simulink model "task1_4"  (R2015b)
settings: Solver=ode45  StartTime=tstart  StopTime=tstop  RelTol=1e-3
values from neighbouring files (symbols this model uses):
  c = 0    [NonLinearAnalysis.m]    (also in Run_Delta_R_Sim.m; analyse_lin_dynamics.m; analyse_steadystate.m; analyse_ulin_dynamics kopi.m)
  delta_max = 0.436332312999    [Yaw and Yaw-rate controller.mat]    (also in Yaw_NonLin_controller.mat; Yaw_PID_controller.mat; run_task1_4.m = deg2rad(25))
  IN = i    [run_task1_4.m]
  K = 0.0516730310612    [Heading_model.mat]    (also in Nomoto2_curvefitting.mat = 0.0627494534487; analyse_controller.m = place(A,B,P); analyse_lin_dynamics.m = x(2); analyse_ulin_dynamics kopi.m = x(2))
  k_b0 = 0.009    [Yaw and Yaw-rate controller.mat]    (also in Yaw_NonLin_controller.mat; Yaw_PID_controller.mat; run_task1_4.m)
  k_b1 = 3.06871796591e-14    [Yaw and Yaw-rate controller.mat]    (also in Yaw_NonLin_controller.mat = 1.2654213265e-10; run_task1_4.m = b_2(2))
  k_b2 = 291.893339409    [Yaw and Yaw-rate controller.mat]    (also in Yaw_NonLin_controller.mat = 288.459058131; run_task1_4.m = b_2(3))
  k_b3 = 1233422.7042    [Yaw and Yaw-rate controller.mat]    (also in Yaw_NonLin_controller.mat = 1209648.75063; run_task1_4.m = b_2(1))
  kd_psi = 3    [Yaw and Yaw-rate controller.mat]    (also in Yaw_NonLin_controller.mat; Yaw_PID_controller.mat = 300; run_task1_4.m = 300)
  ki_psi = 2e-05    [Yaw and Yaw-rate controller.mat]    (also in Yaw_NonLin_controller.mat; Yaw_PID_controller.mat = 0.8; run_task1_4.m = 0.8)
  kp_psi = 0.015    [Yaw and Yaw-rate controller.mat]    (also in Yaw_NonLin_controller.mat; Yaw_PID_controller.mat = 90; run_task1_4.m = 90)
  n_c = 7.3    [run_task1_4.m]
  psi0 = 0    [NonLinearAnalysis.m]    (also in Run_Delta_R_Sim.m; analyse_lin_dynamics.m; analyse_steadystate.m; analyse_ulin_dynamics kopi.m)
  r0 = 0    [NonLinearAnalysis.m]    (also in Run_Delta_R_Sim.m; analyse_lin_dynamics.m; analyse_steadystate.m; analyse_ulin_dynamics kopi.m)
  T1 = 147.34337747    [Heading_model.mat]    (also in Nomoto2_curvefitting.mat = 53.2599278148; analyse_controller.m = 130; analyse_lin_dynamics.m = x(1); analyse_ulin_dynamics kopi.m = x(1))
  T2 = 157.062217136    [Heading_model.mat]    (also in Nomoto2_curvefitting.mat = 67.2891048935; analyse_controller.m = 150; analyse_lin_dynamics.m = x(2); analyse_ulin_dynamics kopi.m = x(2))
  T3 = 252.073612676    [Heading_model.mat]    (also in Nomoto2_curvefitting.mat = 168; analyse_controller.m = 320; analyse_lin_dynamics.m = x(3); analyse_ulin_dynamics kopi.m = x(3))
  tsamp = 10    [NonLinearAnalysis.m]    (also in analyse_lin_dynamics.m; analyse_steadystate.m; analyse_ulin_dynamics kopi.m; analyse_ulin_dynamics.m)
  v0 = [6.63 0]'    [NonLinearAnalysis.m]    (also in Run_Delta_R_Sim.m; analyse_lin_dynamics.m; analyse_steadystate.m; analyse_ulin_dynamics kopi.m)
  w_psi = 0.04    [Yaw and Yaw-rate controller.mat]    (also in Yaw_NonLin_controller.mat; Yaw_PID_controller.mat = 0.05; run_task1_4.m = 0.05)
undefined symbols (not defined in the file or in its folder): msfartoystyring
undefined symbols (not defined in the file): p0
settings Model: ExtModeAutoUpdateStatusClock=off  Creator=christh  LastModifiedBy=Erik
settings DataIOCC: SaveFormat=Array  SignalLoggingSaveFormat=ModelDataLogs
settings OptimizationCC: ExpressionDepthLimit=2147483647  InitFltsAndDblsToZero=on
settings DebuggingCC: UnderspecifiedInitializationDetection=Classic  MergeDetectMultiDrivingBlocksExec=none  SolverPrmCheckMsg=warning  FcnCallInpInsideContextMsg=UseLocalSettings  StateNameClashWarn=warning
settings HardwareCC: ProdBitPerPointer=32  ProdLargestAtomicFloat=None  ProdIntDivRoundTo=Undefined  ProdEndianess=Unspecified  ProdWordSize=32  ProdHWDeviceType=32-bit Generic
settings GRTTargetCC: GeneratePreprocessorConditionals=Disable all  CombineOutputUpdateFcns=off  GRTInterface=on
settings ConfigComp: CovModelRefEnable=Off

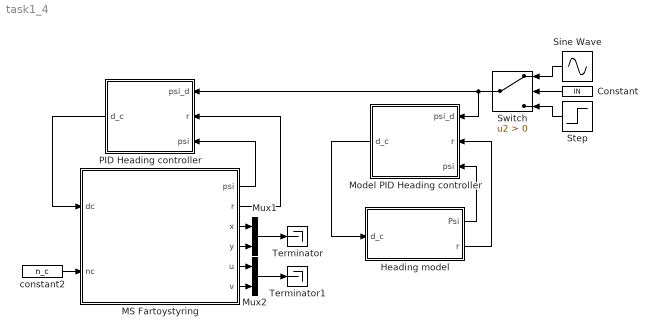
== system task1_4 ==
  Constant : Constant  Value=IN
  Heading model : Subsystem
  MS Fartoystyring : Subsystem  mask(MS Fartoystyring for Assignment 3 G&C){x0=p0(1), y0=p0(2), u0=v0(1), v0=v0(2), psi0=psi0, r0=r0, c=c}
      mask prompts: x0 "x(t0) (m)"; y0 "y(t0) (m)"; u0 "u(t0) (m/s)"; v0 "v(t0) (m/s)"; psi0 "psi(t0) (rad)"; r0 "r(t0) (rad/s)"; c "current (0 or 1)"
      mask help:
      | Block corresponding to Figure 1 in the assignment text. Gives the response of the ship.
      |
      | The design speed of MS Fartoystyring is u=8.23 m/s.
      |
      | Input:
      | dc: commanded rudder (rad), dmax=25*pi/180
      | nc: commanded shaft speed (rad/s), nmax=85*2*pi/60
      |
      | Output:
      | x: north pos (m)
      | y: east pos (m)
      | u: surge (m/s)
      | v: sway (m/s)
      | psi: heading (rad)
      | r: yaw (rad/s)
      mask Help: Comments, bugs and help requests can be directed to the TA. Email on course website.
  Model PID Heading controller : Subsystem
  Mux1 : Mux  Inputs=2
  Mux2 : Mux  Inputs=2
  PID Heading controller : Subsystem
  Sine Wave : Sin  Amplitude=-0.3  Frequency=0.008  SampleTime=0
  Step : Step  Time=20  After=0.3  SampleTime=0
  Switch : Switch  Criteria=u2 > Threshold
  Terminator : Terminator
  Terminator1 : Terminator
  constant2 : Constant  Value=n_c
  wires:
  MS Fartoystyring/1(psi) -> PID Heading controller/3(psi)
  MS Fartoystyring/2(r) -> PID Heading controller/2(r)
  MS Fartoystyring/3(x) -> Mux1/1
  MS Fartoystyring/4(y) -> Mux1/2
  Mux1/1 -> Terminator/1
  constant2/1 -> MS Fartoystyring/2(nc)
  Mux2/1 -> Terminator1/1
  MS Fartoystyring/6(v) -> Mux2/2
  MS Fartoystyring/5(u) -> Mux2/1
  Heading model/1(Psi) -> Model PID Heading controller/3(psi)
  Heading model/2(r) -> Model PID Heading controller/2(r)
  Model PID Heading controller/1(d_c) -> Heading model/1(d_c)
  PID Heading controller/1(d_c) -> MS Fartoystyring/1(dc)
  Switch/1 -> PID Heading controller/1(psi_d), Model PID Heading controller/1(psi_d)
  Constant/1 -> Switch/2
  Sine Wave/1 -> Switch/1
  Step/1 -> Switch/3

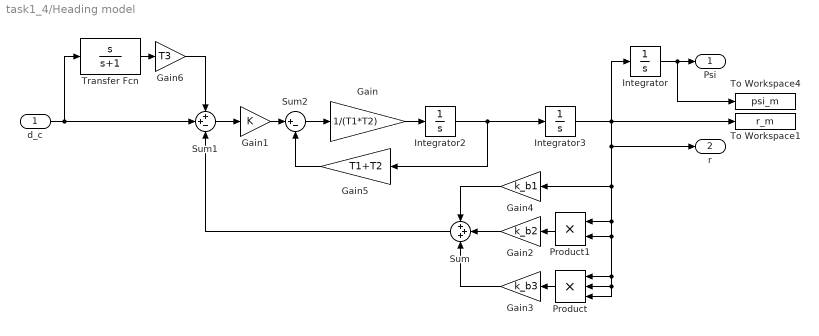
== system task1_4/Heading model ==
  d_c : Inport
  Gain : Gain  Gain=1/(T1*T2)
  Gain1 : Gain  Gain=K
  Gain2 : Gain  Gain=k_b2
  Gain3 : Gain  Gain=k_b3
  Gain4 : Gain  Gain=k_b1
  Gain5 : Gain  Gain=T1+T2
  Gain6 : Gain  Gain=T3
  Integrator : Integrator
  Integrator2 : Integrator
  Integrator3 : Integrator
  Product : Product  Inputs=3
  Product1 : Product
  Sum : Sum  Inputs=+++
  Sum1 : Sum  Inputs=++-
  Sum2 : Sum  Inputs=|+-
  To Workspace1 : ToWorkspace  VariableName=r_m  SampleTime=tsamp
  To Workspace4 : ToWorkspace  VariableName=psi_m  SampleTime=tsamp
  Transfer Fcn : TransferFcn  Numerator=[1 0]  Denominator=[1 1]
  Psi : Outport
  r : Outport  Port=2
  wires:
  Integrator/1 -> To Workspace4/1, Psi/1
  Integrator2/1 -> Gain5/1, Integrator3/1
  Product/1 -> Gain3/1
  Gain/1 -> Integrator2/1
  Sum1/1 -> Gain1/1
  Gain4/1 -> Sum/1
  Gain1/1 -> Sum2/1
  Sum2/1 -> Gain/1
  Gain5/1 -> Sum2/2
  Product1/1 -> Gain2/1
  Integrator3/1 -> r/1, Gain4/1, Product1/1, Product1/2, Product/3, Product/2, Product/1, To Workspace1/1, Integrator/1
  Gain3/1 -> Sum/3
  Gain2/1 -> Sum/2
  d_c/1 -> Transfer Fcn/1, Sum1/2
  Sum/1 -> Sum1/3
  Transfer Fcn/1 -> Gain6/1
  Gain6/1 -> Sum1/1

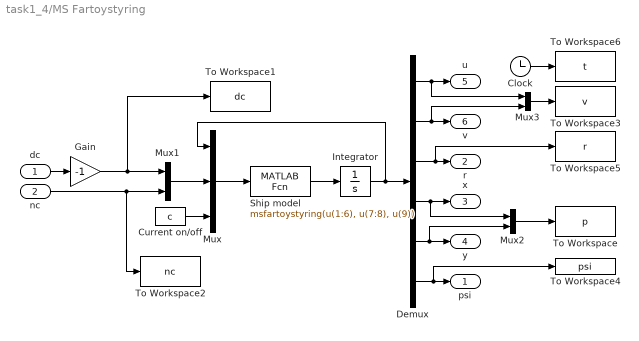
== system task1_4/MS Fartoystyring ==
  dc : Inport
  nc : Inport  Port=2
  Clock : Clock
  Current on/off : Constant  Value=c
  Demux : Demux  Outputs=6
  Gain : Gain  Gain=-1
  Integrator : Integrator  InitialCondition=[u0 v0 r0 x0 y0 psi0]'
  Mux : Mux  Inputs=3
  Mux1 : Mux  Inputs=2
  Mux2 : Mux  Inputs=2
  Mux3 : Mux  Inputs=2
  Ship model : MATLABFcn  MATLABFcn=msfartoystyring(u(1:6), u(7:8), u(9))  OutputDimensions=6
  To Workspace : ToWorkspace  VariableName=p  SampleTime=tsamp
  To Workspace1 : ToWorkspace  VariableName=dc  SampleTime=tsamp
  To Workspace2 : ToWorkspace  VariableName=nc  SampleTime=tsamp
  To Workspace3 : ToWorkspace  VariableName=v  SampleTime=tsamp
  To Workspace4 : ToWorkspace  VariableName=psi  SampleTime=tsamp
  To Workspace5 : ToWorkspace  VariableName=r  SampleTime=tsamp
  To Workspace6 : ToWorkspace  VariableName=t  SampleTime=tsamp
  psi : Outport
  r : Outport  Port=2
  x : Outport  Port=3
  y : Outport  Port=4
  u : Outport  Port=5
  v : Outport  Port=6
  wires:
  Integrator/1 -> Mux/1, Demux/1
  Mux1/1 -> Mux/2
  dc/1 -> Gain/1
  nc/1 -> Mux1/2, To Workspace2/1
  Demux/1 -> Mux3/1, u/1
  Demux/2 -> Mux3/2, v/1
  Demux/3 -> To Workspace5/1, r/1
  Demux/4 -> Mux2/1, x/1
  Demux/5 -> y/1, Mux2/2
  Demux/6 -> To Workspace4/1, psi/1
  Current on/off/1 -> Mux/3
  Ship model/1 -> Integrator/1
  Mux/1 -> Ship model/1
  Mux2/1 -> To Workspace/1
  Clock/1 -> To Workspace6/1
  Mux3/1 -> To Workspace3/1
  Gain/1 -> To Workspace1/1, Mux1/1

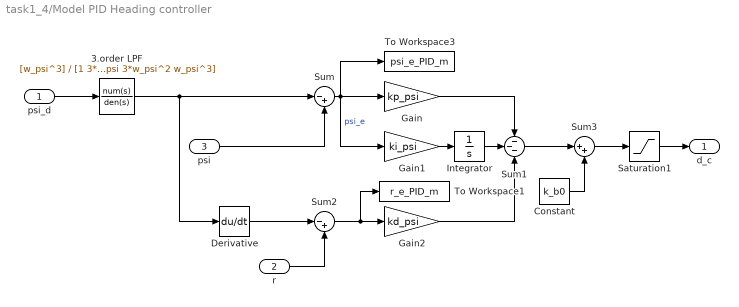
== system task1_4/Model PID Heading controller ==
  psi_d : Inport
  r : Inport  Port=2
  psi : Inport  Port=3
  3.order LPF : TransferFcn  Numerator=[w_psi^3]  Denominator=[1 3*w_psi 3*w_psi^2 w_psi^3]
  Constant : Constant  Value=k_b0
  Derivative : Derivative
  Gain : Gain  Gain=kp_psi
  Gain1 : Gain  Gain=ki_psi
  Gain2 : Gain  Gain=kd_psi
  Integrator : Integrator
  Saturation1 : Saturate  UpperLimit=delta_max  LowerLimit=-delta_max
  Sum : Sum  Inputs=|-+
  Sum1 : Sum  Inputs=---
  Sum2 : Sum  Inputs=|-+
  Sum3 : Sum  Inputs=|++
  To Workspace1 : ToWorkspace  VariableName=r_e_PID_m  SampleTime=tsamp
  To Workspace3 : ToWorkspace  VariableName=psi_e_PID_m  SampleTime=tsamp
  d_c : Outport
  wires:
  psi_d/1 -> 3.order LPF/1
  Saturation1/1 -> d_c/1
  Sum3/1 -> Saturation1/1
  psi/1 -> Sum/2
  Sum/1 -> Gain1/1, Gain/1, To Workspace3/1  "psi_e"
  Gain1/1 -> Integrator/1
  Gain/1 -> Sum1/1
  Integrator/1 -> Sum1/2
  Gain2/1 -> Sum1/3
  Sum1/1 -> Sum3/1
  Constant/1 -> Sum3/2
  Sum2/1 -> To Workspace1/1, Gain2/1
  r/1 -> Sum2/2
  Derivative/1 -> Sum2/1
  3.order LPF/1 -> Derivative/1, Sum/1

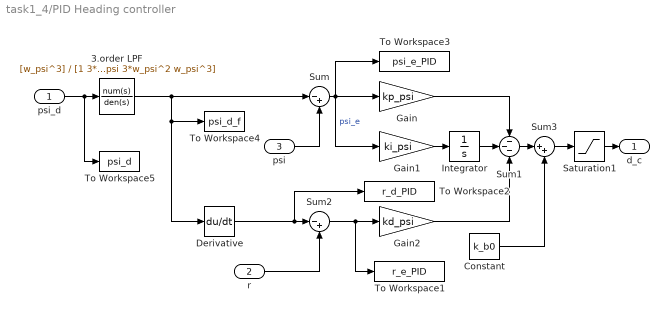
== system task1_4/PID Heading controller ==
  psi_d : Inport
  r : Inport  Port=2
  psi : Inport  Port=3
  3.order LPF : TransferFcn  Numerator=[w_psi^3]  Denominator=[1 3*w_psi 3*w_psi^2 w_psi^3]
  Constant : Constant  Value=k_b0
  Derivative : Derivative
  Gain : Gain  Gain=kp_psi
  Gain1 : Gain  Gain=ki_psi
  Gain2 : Gain  Gain=kd_psi
  Integrator : Integrator
  Saturation1 : Saturate  UpperLimit=delta_max  LowerLimit=-delta_max
  Sum : Sum  Inputs=|-+
  Sum1 : Sum  Inputs=---
  Sum2 : Sum  Inputs=|-+
  Sum3 : Sum  Inputs=|++
  To Workspace1 : ToWorkspace  VariableName=r_e_PID  SampleTime=tsamp
  To Workspace2 : ToWorkspace  VariableName=r_d_PID  SampleTime=tsamp
  To Workspace3 : ToWorkspace  VariableName=psi_e_PID  SampleTime=tsamp
  To Workspace4 : ToWorkspace  VariableName=psi_d_f  SampleTime=tsamp
  To Workspace5 : ToWorkspace  VariableName=psi_d  SampleTime=tsamp
  d_c : Outport
  wires:
  Saturation1/1 -> d_c/1
  Sum3/1 -> Saturation1/1
  psi/1 -> Sum/2
  Sum/1 -> Gain1/1, Gain/1, To Workspace3/1  "psi_e"
  Gain1/1 -> Integrator/1
  Gain/1 -> Sum1/1
  Integrator/1 -> Sum1/2
  Gain2/1 -> Sum1/3
  Sum1/1 -> Sum3/1
  Constant/1 -> Sum3/2
  Sum2/1 -> To Workspace1/1, Gain2/1
  r/1 -> Sum2/2
  Derivative/1 -> To Workspace2/1, Sum2/1
  psi_d/1 -> To Workspace5/1, 3.order LPF/1
  3.order LPF/1 -> Derivative/1, To Workspace4/1, Sum/1
